simulink model "sim_1_simple_model"  (R2022b)
settings: Solver=VariableStepAuto  StartTime=0.0  StopTime=10.0  RelTol=1e-3
libraries: simulink x1
settings Model: Creator=user  LastModifiedBy=user

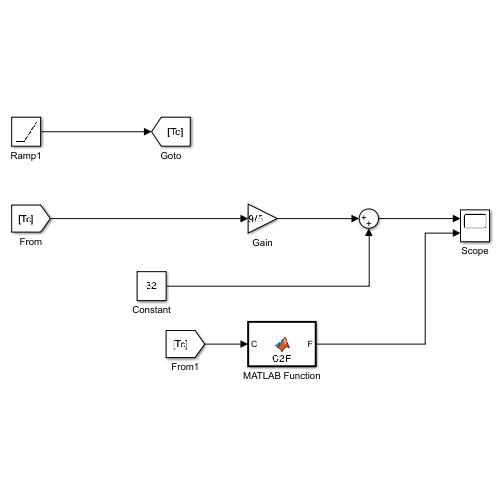
[thumbnail: Simulink's stored preview of the top-level diagram]
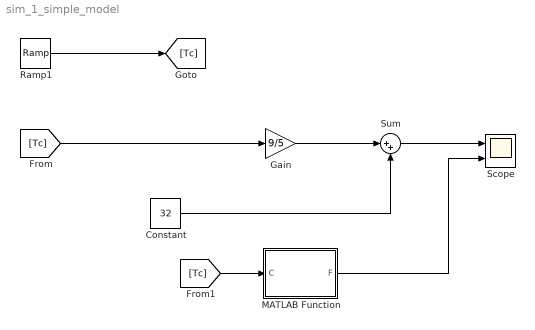
== system sim_1_simple_model ==
  Constant : Constant  Value=32
  Gain : Gain  Gain=9/5
  MATLAB Function : MATLAB Function  TreatAsAtomicUnit=on
  Ramp1 : simulink/Sources/Ramp  slope=1  start=0  InitialOutput=0
  Scope : Scope  NumInputPorts=2
  Sum : Sum  Inputs=|++
  wires:
  Gain/1 -> Sum/1
  Constant/1 -> Sum/2
  Sum/1 -> Scope/1
  Ramp1/1 -> [Tc]
  [Tc] -> Gain/1
  [Tc] -> MATLAB Function/1(C)
  MATLAB Function/1(F) -> Scope/2

== matlab function sim_1_simple_model/MATLAB Function ==
  data: C input; F output
function F = C2F(C)
    F = 9/5 * C + 32;
end
